simulink model "HardwareModel"  (R2023a)
settings: Solver=VariableStepAuto  StartTime=0.0  StopTime=10.0  RelTol=1e-3
model workspace (MAT data in the model file):
  VCO_Input_Voltage = 1
libraries: dspsrcs4 x1, dspxfrm3 x1, dspfdesign x1
settings Model: Creator=Adarsh  LastModifiedBy=Adarsh

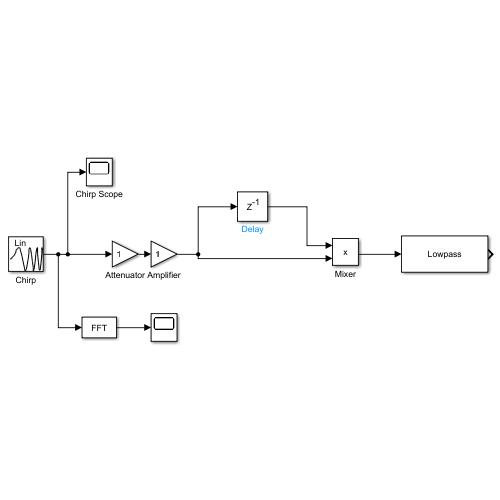
[thumbnail: Simulink's stored preview of the top-level diagram]
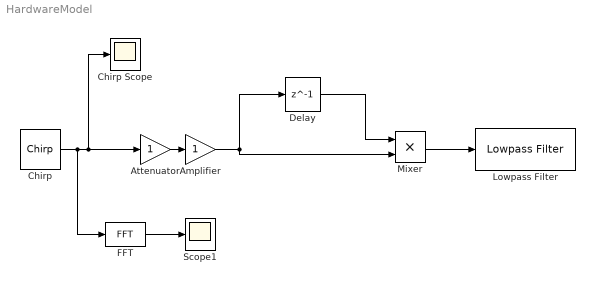
== system HardwareModel ==
  Amplifier : Gain
  Attenuator : Gain
  Chirp : dspsrcs4/Chirp  sweep=Linear  mode=Bidirectional  f0=1000  f1=4000  t1=1  Tsweep=1  phase=0  Ts=1/8000  spf=1  datatype=Double  OutputFrames=off
  Chirp Scope : Scope
  Delay : Delay  DelayLength=1  InitialCondition=0
  FFT : dspxfrm3/FFT  FFTImplementation=Auto  CompMethod=Table lookup  TableOpt=NEW  TableOptActive=Speed  BitRevOrder=off  Normalize=off  InheritFFTLength=on  FFTLength=64  WrapInput=on  roundingMode=Floor  overflowMode=off  firstCoeffDataTypeStr=Inherit: Same word length as input  firstCoeffLastDataTypeStr=Inherit: Same word length as input  outputMin=[]  outputMax=[]
  Lowpass Filter : dspfdesign/Lowpass Filter  FilterType=FIR  DesignForMinimumOrder=on  FilterOrder=50  PassbandFrequency=8e3  StopbandFrequency=12e3  PassbandRipple=0.1  StopbandAttenuation=80  SampleRateMode=Specify on dialog  SampleRate=44100  SimulateUsing=Interpreted execution  roundingMode=Floor  coeffsDataTypeStr=fixdt(1,16)
  Mixer : Product
  Scope1 : Scope
  wires:
  Chirp/1 -> FFT/1, Chirp Scope/1, Attenuator/1
  Attenuator/1 -> Amplifier/1
  Amplifier/1 -> Mixer/2, Delay/1
  Delay/1 -> Mixer/1
  Mixer/1 -> Lowpass Filter/1
  FFT/1 -> Scope1/1
